simulink model "controller"  (R2019a)
settings: Solver=VariableStepAuto  StartTime=0.0  StopTime=2  RelTol=1e-3
values from neighbouring files (symbols this model uses):
  Ke = 17.1e-3    (= 0.0171)    [code.m]    (also in codex.m = 0.05)
  Ta = La/Ra    (= 0.0636428571429)    [code.m]    (also in codex.m = 0.01)
  Tm = J*Ra/(Ke*Km)    (= 0.0197736055538)    [code.m]    (also in codex.m = 0.04)
libraries: fuzblock x1, simulink x1
settings Model: Creator=grove  LastModifiedBy=grove

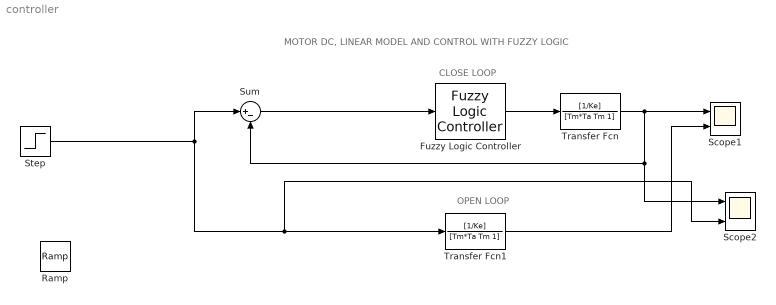
== system controller ==
  note: MOTOR DC, LINEAR MODEL AND CONTROL WITH FUZZY LOGIC
  note: CLOSE LOOP
  note: OPEN LOOP
  Fuzzy Logic Controller : fuzblock/Fuzzy Logic  Controller  FIS=FUZZY4  OutputSampleNumber=101  DataType=double  FuzzifiedInputs=off  RuleFiringStrengths=off  RuleOutputs=off  AggregatedOutputs=off  SimulateUsing=Interpreted execution  OutOfRangeInputValueMessage=warning  NoRuleFiredMessage=warning  EmptyOutputFuzzySetMessage=warning
  Ramp : simulink/Sources/Ramp  slope=5  start=0  InitialOutput=0
  Scope1 : Scope  NumInputPorts=2
  Scope2 : Scope  NumInputPorts=2
  Step : Step  Time=0.1  SampleTime=0
  Sum : Sum  Inputs=|+-
  Transfer Fcn : TransferFcn  Numerator=[1/Ke]  Denominator=[Tm*Ta Tm 1]
  Transfer Fcn1 : TransferFcn  Numerator=[1/Ke]  Denominator=[Tm*Ta Tm 1]
  wires:
  Sum/1 -> Fuzzy Logic Controller/1
  Step/1 -> Sum/1, Scope2/2, Transfer Fcn1/1
  Fuzzy Logic Controller/1 -> Transfer Fcn/1
  Transfer Fcn1/1 -> Scope1/2
  Transfer Fcn/1 -> Scope2/1, Sum/2, Scope1/1
